simulink model "Equaliser"  (R2020a)
settings: Solver=VariableStepAuto  StartTime=0.0  StopTime=100.0  RelTol=1e-3
undefined symbols (not defined in the file): fdesignblkfcn, gcbh
libraries: dspspect3 x1, dspvision x1, dspobslib x1
settings Model: Creator=XPS 15  LastModifiedBy=XPS 15

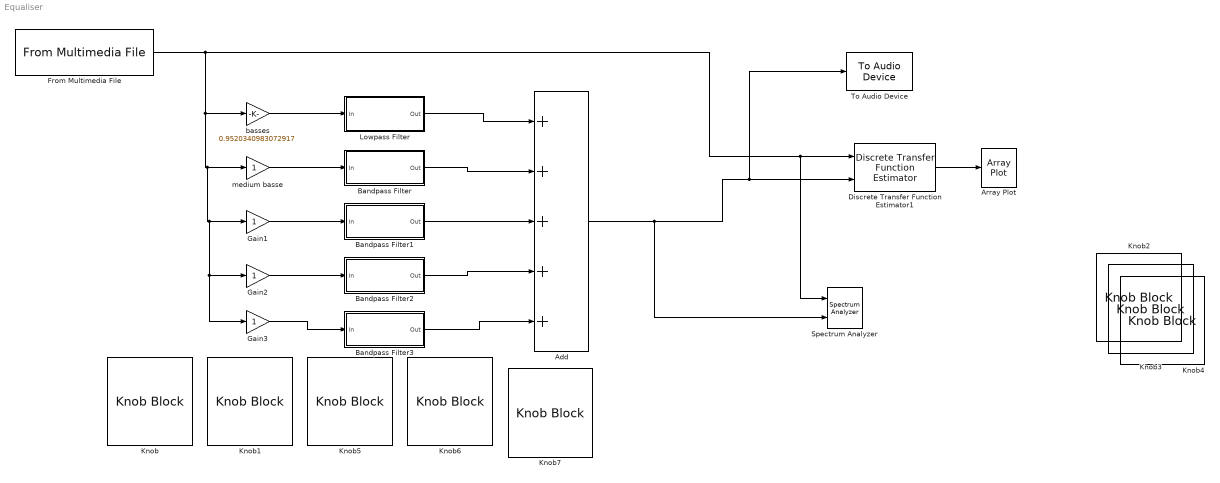
== system Equaliser ==
  Add : Sum  Inputs=+++++
  Array Plot : ArrayPlot
  Bandpass Filter : Subsystem  DialogController=fdesignblkfcn  InitFcn=fdesignblkfcn(gcbh, {'InitFcn'});  mask(Bandpass Filter){}
      mask help: Design a bandpass filter
      settings: CopyFcn=fdesignblkfcn(gcbh, {'CopyFcn'});
      mask Help: helpview(mapfilelocation('dsp'), 'dspbandpassfilter');
      mask Display: disp('Bandpass');
  Bandpass Filter1 : Subsystem  DialogController=fdesignblkfcn  InitFcn=fdesignblkfcn(gcbh, {'InitFcn'});  mask(Bandpass Filter){}
      mask help: Design a bandpass filter
      settings: CopyFcn=fdesignblkfcn(gcbh, {'CopyFcn'});
      mask Help: helpview(mapfilelocation('dsp'), 'dspbandpassfilter');
      mask Display: disp('Bandpass');
  Bandpass Filter2 : Subsystem  DialogController=fdesignblkfcn  InitFcn=fdesignblkfcn(gcbh, {'InitFcn'});  mask(Bandpass Filter){}
      mask help: Design a bandpass filter
      settings: CopyFcn=fdesignblkfcn(gcbh, {'CopyFcn'});
      mask Help: helpview(mapfilelocation('dsp'), 'dspbandpassfilter');
      mask Display: disp('Bandpass');
  Bandpass Filter3 : Subsystem  DialogController=fdesignblkfcn  InitFcn=fdesignblkfcn(gcbh, {'InitFcn'});  mask(Bandpass Filter){}
      mask help: Design a bandpass filter
      settings: CopyFcn=fdesignblkfcn(gcbh, {'CopyFcn'});
      mask Help: helpview(mapfilelocation('dsp'), 'dspbandpassfilter');
      mask Display: disp('Bandpass');
  Discrete Transfer Function Estimator1 : dspspect3/Discrete Transfer Function Estimator  WindowMode=Specify on dialog  WindowLength=1024  Overlap=50  AveragingMethod=Running  ForgettingFactorPort=off  ForgettingFactor=0.9  SpectralAverages=100  FFTLengthSource=Auto  FFTLength=128  Window=Hann  SidelobeAttenuation=60  FrequencyRange=One-sided  OutputCoherence=off  SimulateUsing=Code generation
      settings: SourceProductBaseCode=DS
  From Multimedia File : dspvision/From Multimedia File  inputFilename=C:\Users\XPS 15\Desktop\L05 Sorbonne\images\Son\Projet\guitare.wav  readRange=[1 Inf]  loop=on  numPlays=inf  outputStreams=Audio only  videoDataType=single  audioDataType=double  inheritSampleTime=on  userDefinedSampleTime=1/30  noAudioOutput=off  isIntensityVideo=off  fourcc=RGB  colorVideoFormat=Separate color signals  outputEOF=off  dataOrg=Column-major  audioFrameSize=11025  computeAudioFrameSize=off  outSamplingMode=Sample based
  Gain1 : Gain
  Gain2 : Gain
  Gain3 : Gain
  Knob{,1,5..7} (5 alike) : KnobBlock  ScaleMax=1
  Knob2 : KnobBlock
  Knob3 : KnobBlock
  Knob4 : KnobBlock
  Lowpass Filter : Subsystem  DialogController=fdesignblkfcn  InitFcn=fdesignblkfcn(gcbh, {'InitFcn'});  mask(Lowpass Filter){}
      mask help: Design a lowpass filter
      settings: CopyFcn=fdesignblkfcn(gcbh, {'CopyFcn'});
      mask Help: helpview(mapfilelocation('dsp'), 'dsplowpassfilter');
      mask Display: disp('Lowpass')
  Spectrum Analyzer : SpectrumAnalyzer  NumInputPorts=2
  To Audio Device : dspobslib/To Audio Device  deviceName=Default  inheritSampleRate=on  sampleRate=44100  deviceDatatype=Determine from input data type  autoBufferSize=on  bufferSize=4096  queueDuration=1.0  defaultOutputChannelMapping=on  outputChannelMapping=1:2  outputNumUnderrunSamples=off
      settings: SourceProductBaseCode=DS
  basses : Gain  Gain=0.9520340983072917
  medium basse : Gain
  wires:
  From Multimedia File/1 -> Gain3/1, Gain2/1, Gain1/1, medium basse/1, basses/1, Spectrum Analyzer/1, Discrete Transfer Function Estimator1/1
  Discrete Transfer Function Estimator1/1 -> Array Plot/1
  Bandpass Filter2/1(Out) -> Add/4
  Lowpass Filter/1(Out) -> Add/1
  Bandpass Filter/1(Out) -> Add/2
  Bandpass Filter1/1(Out) -> Add/3
  Add/1 -> Spectrum Analyzer/2, To Audio Device/1, Discrete Transfer Function Estimator1/2
  basses/1 -> Lowpass Filter/1(In)
  medium basse/1 -> Bandpass Filter/1(In)
  Gain1/1 -> Bandpass Filter1/1(In)
  Gain2/1 -> Bandpass Filter2/1(In)
  Gain3/1 -> Bandpass Filter3/1(In)
  Bandpass Filter3/1(Out) -> Add/5

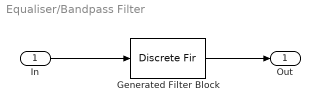
== system Equaliser/Bandpass Filter ==
  In : Inport
  Generated Filter Block : DiscreteFir  Tag=BlockMethodSubSystem  Coefficients=[0.0203951895353563437 0.0105270395880383734 0.00102609416191840616 -0.00105638581872127693 0.0103630090032638365 0.019415288736150612 0.00983620951138712736 -0.00777295666343813963 -0.00799308481954388687 0.00992847112640252161 0.0156072059452413477 -0.00813260066507140444 -0.0338743714257357525 -0.0259768787159957264 0.00154804325119133881 -0.00212638512934792707 -0.0472890105468602717 -0.076238130825818165 -0.0433792974890072763 0.00370068499008208629 -0.0239510735780798616 -0.118018766943639497 -0.143446554112368119 0.00585984642262463336 0.24727995264986749 0.366139803324822433 0.24727995264986749 0.00585984642262463336 -0.143446554112368119 -0.118018766943639497 -0.0239510735780798616 0.00370068499008208629 -0.0433792974890072763 -0.076238130825818165 -0.0472890105468602717 -0.00212638512934792707 0.00154804325119133881 -0.0259768787159957264 -0.0338743714257357525 -0.00813260066507140444 0.0156072059452413477 0.00992847112640252161 -0.00799308481954388687 -0.00777295666343813963 0.00983620951138712736 0.019415288736150612 0.0103630090032638365 -0.00105638581872127693 0.00102609416191840616 0.0105270395880383734 0.0203951895353563437]  InputProcessing=Columns as channels (frame based)
  Out : Outport
  wires:
  Generated Filter Block/1 -> Out/1
  In/1 -> Generated Filter Block/1

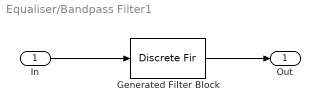
== system Equaliser/Bandpass Filter1 ==
  In : Inport
  Generated Filter Block : DiscreteFir  Tag=BlockMethodSubSystem  Coefficients=[0.00135877272117858848 0.00509218721067843973 -0.00107535442758440879 0.000709082871088827249 0.000222922703759563474 -0.00846638313535847536 -0.00454201081853635846 0.0137730039030066424 0.0095749613740041227 -0.00837718850712794449 -0.00338280231013474977 -0.00341278122921825043 -0.0196864163133547675 0.00632288751786394716 0.0433596688516629664 0.00486449262220048015 -0.0375113620465250541 -0.00772055466820894404 -0.00938074169701247872 -0.0333704038935819097 0.0673859704006575244 0.126474928606283954 -0.0849038664324290315 -0.22862219075809434 0.0385802579943139989 0.273354590512590645 0.0385802579943139989 -0.22862219075809434 -0.0849038664324290315 0.126474928606283954 0.0673859704006575244 -0.0333704038935819097 -0.00938074169701247872 -0.00772055466820894404 -0.0375113620465250541 0.00486449262220048015 0.0433596688516629664 0.00632288751786394716 -0.0196864163133547675 -0.00341278122921825043 -0.00338280231013474977 -0.00837718850712794449 0.0095749613740041227 0.0137730039030066424 -0.00454201081853635846 -0.00846638313535847536 0.000222922703759563474 0.000709082871088827249 -0.00107535442758440879 0.00509218721067843973 0.00135877272117858848]  InputProcessing=Columns as channels (frame based)
  Out : Outport
  wires:
  Generated Filter Block/1 -> Out/1
  In/1 -> Generated Filter Block/1

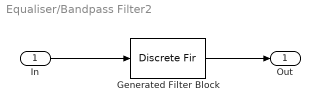
== system Equaliser/Bandpass Filter2 ==
  In : Inport
  Generated Filter Block : DiscreteFir  Tag=BlockMethodSubSystem  Coefficients=[0.00099985025894186539 -0.00689822537468701927 0.00679631455291792447 -0.00532269753112438702 0.00203354292113842698 -0.00177505112775096295 0.00740645273183580203 -0.0163789916372325157 0.021590209858332321 -0.017819304154848066 0.00813318651443768574 -0.00316427909481966415 0.0118405613274002695 -0.0311071986721033616 0.0455113754877628229 -0.0398870549286385601 0.0156089237811597378 0.00559365238182654885 0.00228146665188617981 -0.0439220412312785885 0.0899637344990159016 -0.0923794146506985575 0.0206924028811565457 0.108231784323620975 -0.232858021465985332 0.284346942980266304 -0.232858021465985332 0.108231784323620975 0.0206924028811565457 -0.0923794146506985575 0.0899637344990159016 -0.0439220412312785885 0.00228146665188617981 0.00559365238182654885 0.0156089237811597378 -0.0398870549286385601 0.0455113754877628229 -0.0311071986721033616 0.0118405613274002695 -0.00316427909481966415 0.00813318651443768574 -0.017819304154848066 0.021590209858332321 -0.0163789916372325157 0.00740645273183580203 -0.00177505112775096295 0.00203354292113842698 -0.00532269753112438702 0.00679631455291792447 -0.00689822537468701927 0.00099985025894186539]  InputProcessing=Columns as channels (frame based)
  Out : Outport
  wires:
  Generated Filter Block/1 -> Out/1
  In/1 -> Generated Filter Block/1

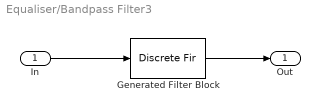
== system Equaliser/Bandpass Filter3 ==
  In : Inport
  Generated Filter Block : DiscreteFir  Tag=BlockMethodSubSystem  Coefficients=[-0.00375672239269892903 0.00391580605713855862 0.00181116792460870538 0.00103291782042095183 -0.00162250139777729736 -0.00494051707968386992 0.0133720527368652049 -0.00334940143374779647 -0.0128223380434725164 0.0108460428469768361 0.000355528521909860844 0.00710741211822148514 -0.0146546247891593644 -0.0126887099016466387 0.0437597799111126423 -0.020936068437688915 -0.024343302492758543 0.0192295475289383233 0.00191329935289041549 0.0434629922595457449 -0.0861446300376062929 -0.0190929314106859163 0.190948244955503804 -0.157907186640566133 -0.108815954249417438 0.273283445577948481 -0.108815954249417438 -0.157907186640566133 0.190948244955503804 -0.0190929314106859163 -0.0861446300376062929 0.0434629922595457449 0.00191329935289041549 0.0192295475289383233 -0.024343302492758543 -0.020936068437688915 0.0437597799111126423 -0.0126887099016466387 -0.0146546247891593644 0.00710741211822148514 0.000355528521909860844 0.0108460428469768361 -0.0128223380434725164 -0.00334940143374779647 0.0133720527368652049 -0.00494051707968386992 -0.00162250139777729736 0.00103291782042095183 0.00181116792460870538 0.00391580605713855862 -0.00375672239269892903]  InputProcessing=Columns as channels (frame based)
  Out : Outport
  wires:
  Generated Filter Block/1 -> Out/1
  In/1 -> Generated Filter Block/1

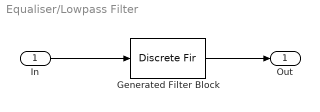
== system Equaliser/Lowpass Filter ==
  In : Inport
  Generated Filter Block : DiscreteFir  Tag=BlockMethodSubSystem  Coefficients=[0.0740309425242378499 0.124494427598271798 -0.093660668811036546 0.00353679654821630876 -0.0378371530414057661 -0.0188276332392776184 -0.0262748234084314511 -0.0215713453365450232 -0.0214622703311879263 -0.0183611187364709147 -0.0152012772330087659 -0.0105485338068202171 -0.00502574439809432092 0.00162565823437747542 0.00915466087540308705 0.0174276643141721595 0.0263462007241276955 0.0355335578879064085 0.0446937311668279755 0.053639583934940907 0.0617260422936317873 0.0686348042911524708 0.0745806601326779867 0.0790514574903630474 0.0817954229985850545 0.0824990424393100136 0.0817954229985850545 0.0790514574903630474 0.0745806601326779867 0.0686348042911524708 0.0617260422936317873 0.053639583934940907 0.0446937311668279755 0.0355335578879064085 0.0263462007241276955 0.0174276643141721595 0.00915466087540308705 0.00162565823437747542 -0.00502574439809432092 -0.0105485338068202171 -0.0152012772330087659 -0.0183611187364709147 -0.0214622703311879263 -0.0215713453365450232 -0.0262748234084314511 -0.0188276332392776184 -0.0378371530414057661 0.00353679654821630876 -0.093660668811036546 0.124494427598271798 0.0740309425242378499]  InputProcessing=Columns as channels (frame based)
  Out : Outport
  wires:
  Generated Filter Block/1 -> Out/1
  In/1 -> Generated Filter Block/1
